simulink model "Brown_Control_Sim"  (R2025b)
settings: Solver=VariableStepAuto  StartTime=0.0  StopTime=10  RelTol=1e-3
undefined symbols (not defined in the file or in its folder): controller_airspeed_cmd_base, controller_airspeed_step, controller_bank_cmd_base, controller_bank_step, controller_enable, controller_front_motor_mask, controller_integrator_limit, controller_k_p_damp, controller_k_phi_i, controller_k_phi_p, controller_k_q_damp, controller_k_r_damp, controller_k_v_i, controller_k_v_p, controller_mode, controller_rpm_delta_limit, controller_sample_time, controller_step_time, controller_surface_limit_rad, controller_trim_delta_a, controller_trim_delta_e, controller_trim_delta_f, controller_trim_delta_r, controller_trim_motor_rpms, controller_trim_tilt_angles, estimator_enable, estimator_init_eul, estimator_k_acc, estimator_k_att, estimator_k_mag, estimator_sample_time, mag_ned, sensor_accel_bias, sensor_accel_sigma, sensor_airdata_bias, sensor_airdata_sigma, sensor_attitude_bias, sensor_attitude_sigma, sensor_enable_bias, sensor_enable_noise, sensor_gps_pos_bias, sensor_gps_pos_sigma, sensor_gps_vel_bias, sensor_gps_vel_sigma, sensor_gyro_bias, sensor_gyro_sigma, sensor_mag_bias, sensor_mag_sigma, sensor_sample_time, trim_front_collective_rpm, trim_rear_collective_rpm
settings Model: Creator=zbrown  LastModifiedBy=zbrown

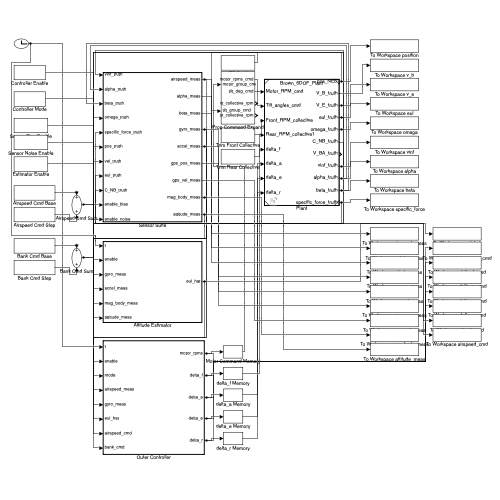
[thumbnail: Simulink's stored preview of the top-level diagram]
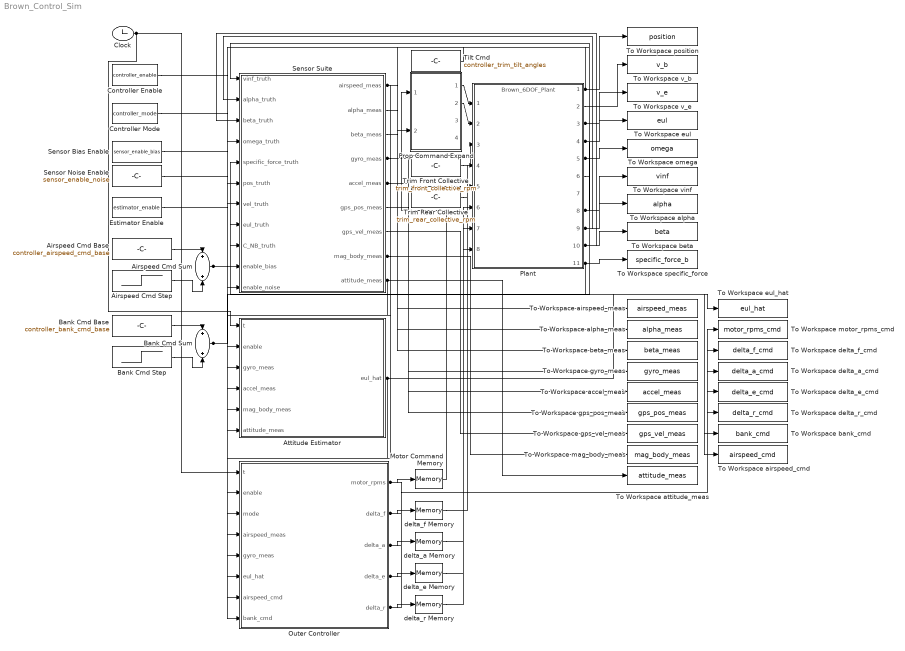
== system Brown_Control_Sim ==
  Airspeed Cmd Base : Constant  Value=controller_airspeed_cmd_base
  Airspeed Cmd Step : Step  Time=controller_step_time  After=controller_airspeed_step  SampleTime=0
  Airspeed Cmd Sum : Sum
  Attitude Estimator : Subsystem  TreatAsAtomicUnit=on  SystemSampleTime=estimator_sample_time
  Bank Cmd Base : Constant  Value=controller_bank_cmd_base
  Bank Cmd Step : Step  Time=controller_step_time  After=controller_bank_step  SampleTime=0
  Bank Cmd Sum : Sum
  Clock : Clock
  Controller Enable : Constant  Value=controller_enable
  Controller Mode : Constant  Value=controller_mode
  Estimator Enable : Constant  Value=estimator_enable
  Motor Command Memory : Memory
  Outer Controller : Subsystem  TreatAsAtomicUnit=on  SystemSampleTime=controller_sample_time
  Plant : ModelReference  ModelNameDialog=Brown_6DOF_Plant  SimulationMode=Normal  ModelReferenceVersion=1.27
  Prop Command Expand : Subsystem
  Sensor Bias Enable : Constant  Value=sensor_enable_bias
  Sensor Noise Enable : Constant  Value=sensor_enable_noise
  Sensor Suite : Subsystem  TreatAsAtomicUnit=on  SystemSampleTime=sensor_sample_time
  Tilt Cmd : Constant  Value=controller_trim_tilt_angles
  To Workspace accel_meas : ToWorkspace  VariableName=accel_meas  SampleTime=-1
  To Workspace airspeed_cmd : ToWorkspace  VariableName=airspeed_cmd  SampleTime=-1
  To Workspace airspeed_meas : ToWorkspace  VariableName=airspeed_meas  SampleTime=-1
  To Workspace alpha : ToWorkspace  VariableName=alpha  SampleTime=-1
  To Workspace alpha_meas : ToWorkspace  VariableName=alpha_meas  SampleTime=-1
  To Workspace attitude_meas : ToWorkspace  VariableName=attitude_meas  SampleTime=-1
  To Workspace bank_cmd : ToWorkspace  VariableName=bank_cmd  SampleTime=-1
  To Workspace beta : ToWorkspace  VariableName=beta  SampleTime=-1
  To Workspace beta_meas : ToWorkspace  VariableName=beta_meas  SampleTime=-1
  To Workspace delta_a_cmd : ToWorkspace  VariableName=delta_a_cmd  SampleTime=-1
  To Workspace delta_e_cmd : ToWorkspace  VariableName=delta_e_cmd  SampleTime=-1
  To Workspace delta_f_cmd : ToWorkspace  VariableName=delta_f_cmd  SampleTime=-1
  To Workspace delta_r_cmd : ToWorkspace  VariableName=delta_r_cmd  SampleTime=-1
  To Workspace eul : ToWorkspace  VariableName=eul  SampleTime=-1
  To Workspace eul_hat : ToWorkspace  VariableName=eul_hat  SampleTime=-1
  To Workspace gps_pos_meas : ToWorkspace  VariableName=gps_pos_meas  SampleTime=-1
  To Workspace gps_vel_meas : ToWorkspace  VariableName=gps_vel_meas  SampleTime=-1
  To Workspace gyro_meas : ToWorkspace  VariableName=gyro_meas  SampleTime=-1
  To Workspace mag_body_meas : ToWorkspace  VariableName=mag_body_meas  SampleTime=-1
  To Workspace motor_rpms_cmd : ToWorkspace  VariableName=motor_rpms_cmd  SampleTime=-1
  To Workspace omega : ToWorkspace  VariableName=omega  SampleTime=-1
  To Workspace position : ToWorkspace  VariableName=position  SampleTime=-1
  To Workspace specific_force : ToWorkspace  VariableName=specific_force_b  SampleTime=-1
  To Workspace v_b : ToWorkspace  VariableName=v_b  SampleTime=-1
  To Workspace v_e : ToWorkspace  VariableName=v_e  SampleTime=-1
  To Workspace vinf : ToWorkspace  VariableName=vinf  SampleTime=-1
  Trim Front Collective : Constant  Value=trim_front_collective_rpm
  Trim Rear Collective : Constant  Value=trim_rear_collective_rpm
  delta_a Memory : Memory
  delta_e Memory : Memory
  delta_f Memory : Memory
  delta_r Memory : Memory
  wires:
  Airspeed Cmd Base/1 -> Airspeed Cmd Sum/1
  Airspeed Cmd Step/1 -> Airspeed Cmd Sum/2
  Bank Cmd Base/1 -> Bank Cmd Sum/1
  Bank Cmd Step/1 -> Bank Cmd Sum/2
  Outer Controller/1(motor_rpms) -> Motor Command Memory/1, To Workspace motor_rpms_cmd/1
  Outer Controller/2(delta_f) -> delta_f Memory/1, To Workspace delta_f_cmd/1
  Outer Controller/3(delta_a) -> delta_a Memory/1, To Workspace delta_a_cmd/1
  Outer Controller/4(delta_e) -> delta_e Memory/1, To Workspace delta_e_cmd/1
  Outer Controller/5(delta_r) -> delta_r Memory/1, To Workspace delta_r_cmd/1
  Motor Command Memory/1 -> Prop Command Expand/1(motor_group_cmd)
  Tilt Cmd/1 -> Prop Command Expand/2(tilt_group_cmd)
  Prop Command Expand/1(motor_rpms_cmd) -> Plant/1
  Prop Command Expand/2(tilt_deg_cmd) -> Plant/2
  Trim Front Collective/1 -> Plant/3
  Trim Rear Collective/1 -> Plant/4
  delta_f Memory/1 -> Plant/5
  delta_a Memory/1 -> Plant/6
  delta_e Memory/1 -> Plant/7
  delta_r Memory/1 -> Plant/8
  Plant/8 -> Sensor Suite/1(vinf_truth), To Workspace vinf/1
  Plant/9 -> Sensor Suite/2(alpha_truth), To Workspace alpha/1
  Plant/10 -> Sensor Suite/3(beta_truth), To Workspace beta/1
  Plant/5 -> Sensor Suite/4(omega_truth), To Workspace omega/1
  Plant/11 -> Sensor Suite/5(specific_force_truth), To Workspace specific_force/1
  Plant/1 -> Sensor Suite/6(pos_truth), To Workspace position/1
  Plant/3 -> Sensor Suite/7(vel_truth), To Workspace v_e/1
  Plant/4 -> Sensor Suite/8(eul_truth), To Workspace eul/1
  Plant/6 -> Sensor Suite/9(C_NB_truth)
  Sensor Bias Enable/1 -> Sensor Suite/10(enable_bias)
  Sensor Noise Enable/1 -> Sensor Suite/11(enable_noise)
  Clock/1 -> Attitude Estimator/1(t), Outer Controller/1(t)
  Estimator Enable/1 -> Attitude Estimator/2(enable)
  Sensor Suite/4(gyro_meas) -> Attitude Estimator/3(gyro_meas), Outer Controller/5(gyro_meas), To Workspace gyro_meas/1
  Sensor Suite/5(accel_meas) -> Attitude Estimator/4(accel_meas), To Workspace accel_meas/1
  Sensor Suite/8(mag_body_meas) -> Attitude Estimator/5(mag_body_meas), To Workspace mag_body_meas/1
  Sensor Suite/9(attitude_meas) -> Attitude Estimator/6(attitude_meas), To Workspace attitude_meas/1
  Controller Enable/1 -> Outer Controller/2(enable)
  Controller Mode/1 -> Outer Controller/3(mode)
  Sensor Suite/1(airspeed_meas) -> Outer Controller/4(airspeed_meas), To Workspace airspeed_meas/1
  Attitude Estimator/1(eul_hat) -> Outer Controller/6(eul_hat), To Workspace eul_hat/1
  Airspeed Cmd Sum/1 -> Outer Controller/7(airspeed_cmd), To Workspace airspeed_cmd/1
  Bank Cmd Sum/1 -> Outer Controller/8(bank_cmd), To Workspace bank_cmd/1
  Plant/2 -> To Workspace v_b/1
  Sensor Suite/2(alpha_meas) -> To Workspace alpha_meas/1
  Sensor Suite/3(beta_meas) -> To Workspace beta_meas/1
  Sensor Suite/6(gps_pos_meas) -> To Workspace gps_pos_meas/1
  Sensor Suite/7(gps_vel_meas) -> To Workspace gps_vel_meas/1

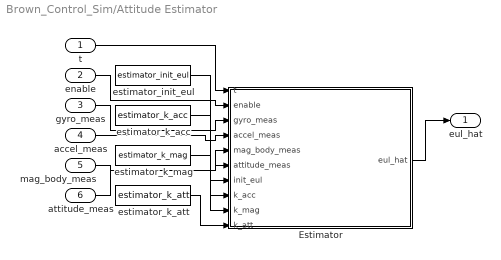
== system Brown_Control_Sim/Attitude Estimator ==
  t : Inport
  enable : Inport  Port=2
  gyro_meas : Inport  Port=3
  accel_meas : Inport  Port=4
  mag_body_meas : Inport  Port=5
  attitude_meas : Inport  Port=6
  Estimator : MATLAB Function  TreatAsAtomicUnit=on
  estimator_init_eul : Constant  Value=estimator_init_eul
  estimator_k_acc : Constant  Value=estimator_k_acc
  estimator_k_att : Constant  Value=estimator_k_att
  estimator_k_mag : Constant  Value=estimator_k_mag
  eul_hat : Outport
  wires:
  ? -> ?
  t/1 -> Estimator/1(t)
  enable/1 -> Estimator/2(enable)
  gyro_meas/1 -> Estimator/3(gyro_meas)
  accel_meas/1 -> Estimator/4(accel_meas)
  mag_body_meas/1 -> Estimator/5(mag_body_meas)
  attitude_meas/1 -> Estimator/6(attitude_meas)
  estimator_init_eul/1 -> Estimator/7(init_eul)
  estimator_k_acc/1 -> Estimator/8(k_acc)
  estimator_k_mag/1 -> Estimator/9(k_mag)
  estimator_k_att/1 -> Estimator/10(k_att)
  Estimator/1(eul_hat) -> eul_hat/1

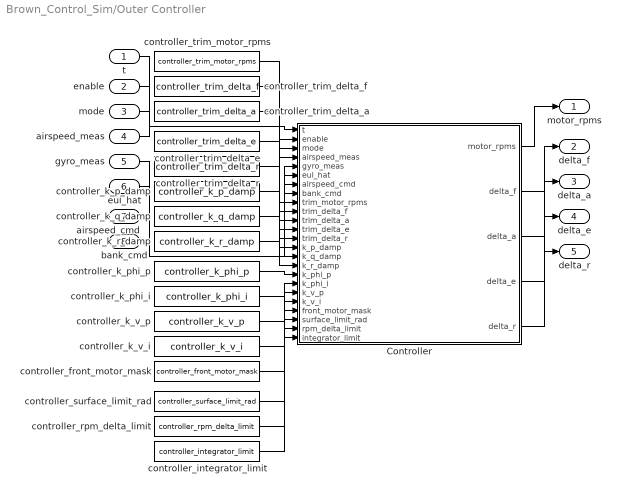
== system Brown_Control_Sim/Outer Controller ==
  t : Inport
  enable : Inport  Port=2
  mode : Inport  Port=3
  airspeed_meas : Inport  Port=4
  gyro_meas : Inport  Port=5
  eul_hat : Inport  Port=6
  airspeed_cmd : Inport  Port=7
  bank_cmd : Inport  Port=8
  Controller : MATLAB Function  TreatAsAtomicUnit=on
  controller_front_motor_mask : Constant  Value=controller_front_motor_mask
  controller_integrator_limit : Constant  Value=controller_integrator_limit
  controller_k_p_damp : Constant  Value=controller_k_p_damp
  controller_k_phi_i : Constant  Value=controller_k_phi_i
  controller_k_phi_p : Constant  Value=controller_k_phi_p
  controller_k_q_damp : Constant  Value=controller_k_q_damp
  controller_k_r_damp : Constant  Value=controller_k_r_damp
  controller_k_v_i : Constant  Value=controller_k_v_i
  controller_k_v_p : Constant  Value=controller_k_v_p
  controller_rpm_delta_limit : Constant  Value=controller_rpm_delta_limit
  controller_surface_limit_rad : Constant  Value=controller_surface_limit_rad
  controller_trim_delta_a : Constant  Value=controller_trim_delta_a
  controller_trim_delta_e : Constant  Value=controller_trim_delta_e
  controller_trim_delta_f : Constant  Value=controller_trim_delta_f
  controller_trim_delta_r : Constant  Value=controller_trim_delta_r
  controller_trim_motor_rpms : Constant  Value=controller_trim_motor_rpms
  motor_rpms : Outport
  delta_f : Outport  Port=2
  delta_a : Outport  Port=3
  delta_e : Outport  Port=4
  delta_r : Outport  Port=5
  wires:
  ? -> ?
  t/1 -> Controller/1(t)
  enable/1 -> Controller/2(enable)
  mode/1 -> Controller/3(mode)
  airspeed_meas/1 -> Controller/4(airspeed_meas)
  gyro_meas/1 -> Controller/5(gyro_meas)
  eul_hat/1 -> Controller/6(eul_hat)
  airspeed_cmd/1 -> Controller/7(airspeed_cmd)
  bank_cmd/1 -> Controller/8(bank_cmd)
  controller_trim_motor_rpms/1 -> Controller/9(trim_motor_rpms)
  controller_trim_delta_f/1 -> Controller/10(trim_delta_f)
  controller_trim_delta_a/1 -> Controller/11(trim_delta_a)
  controller_trim_delta_e/1 -> Controller/12(trim_delta_e)
  controller_trim_delta_r/1 -> Controller/13(trim_delta_r)
  controller_k_p_damp/1 -> Controller/14(k_p_damp)
  controller_k_q_damp/1 -> Controller/15(k_q_damp)
  controller_k_r_damp/1 -> Controller/16(k_r_damp)
  controller_k_phi_p/1 -> Controller/17(k_phi_p)
  controller_k_phi_i/1 -> Controller/18(k_phi_i)
  controller_k_v_p/1 -> Controller/19(k_v_p)
  controller_k_v_i/1 -> Controller/20(k_v_i)
  controller_front_motor_mask/1 -> Controller/21(front_motor_mask)
  controller_surface_limit_rad/1 -> Controller/22(surface_limit_rad)
  controller_rpm_delta_limit/1 -> Controller/23(rpm_delta_limit)
  controller_integrator_limit/1 -> Controller/24(integrator_limit)
  Controller/1(motor_rpms) -> motor_rpms/1
  Controller/2(delta_f) -> delta_f/1
  Controller/3(delta_a) -> delta_a/1
  Controller/4(delta_e) -> delta_e/1
  Controller/5(delta_r) -> delta_r/1

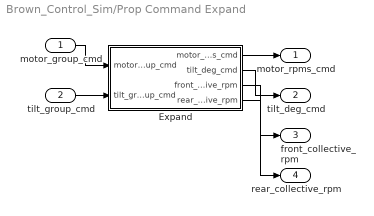
== system Brown_Control_Sim/Prop Command Expand ==
  motor_group_cmd : Inport
  tilt_group_cmd : Inport  Port=2
  Expand : MATLAB Function  TreatAsAtomicUnit=on
  motor_rpms_cmd : Outport
  tilt_deg_cmd : Outport  Port=2
  front_collective_rpm : Outport  Port=3
  rear_collective_rpm : Outport  Port=4
  wires:
  ? -> ?
  motor_group_cmd/1 -> Expand/1(motor_group_cmd)
  tilt_group_cmd/1 -> Expand/2(tilt_group_cmd)
  Expand/1(motor_rpms_cmd) -> motor_rpms_cmd/1
  Expand/2(tilt_deg_cmd) -> tilt_deg_cmd/1
  Expand/3(front_collective_rpm) -> front_collective_rpm/1
  Expand/4(rear_collective_rpm) -> rear_collective_rpm/1

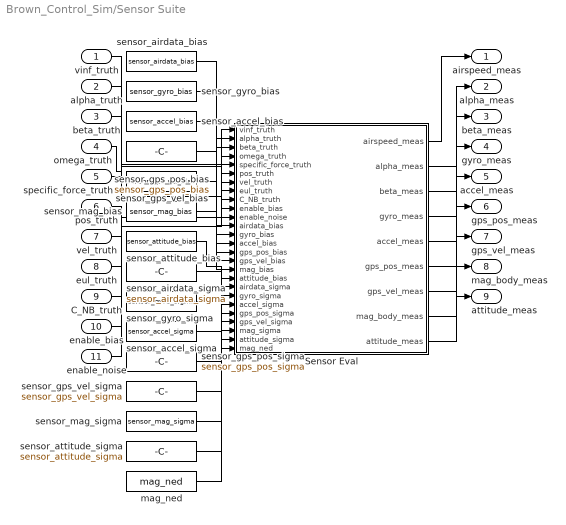
== system Brown_Control_Sim/Sensor Suite ==
  vinf_truth : Inport
  alpha_truth : Inport  Port=2
  beta_truth : Inport  Port=3
  omega_truth : Inport  Port=4
  specific_force_truth : Inport  Port=5
  pos_truth : Inport  Port=6
  vel_truth : Inport  Port=7
  eul_truth : Inport  Port=8
  C_NB_truth : Inport  Port=9
  enable_bias : Inport  Port=10
  enable_noise : Inport  Port=11
  Sensor Eval : MATLAB Function  TreatAsAtomicUnit=on
  mag_ned : Constant  Value=mag_ned
  sensor_accel_bias : Constant  Value=sensor_accel_bias
  sensor_accel_sigma : Constant  Value=sensor_accel_sigma
  sensor_airdata_bias : Constant  Value=sensor_airdata_bias
  sensor_airdata_sigma : Constant  Value=sensor_airdata_sigma
  sensor_attitude_bias : Constant  Value=sensor_attitude_bias
  sensor_attitude_sigma : Constant  Value=sensor_attitude_sigma
  sensor_gps_pos_bias : Constant  Value=sensor_gps_pos_bias
  sensor_gps_pos_sigma : Constant  Value=sensor_gps_pos_sigma
  sensor_gps_vel_bias : Constant  Value=sensor_gps_vel_bias
  sensor_gps_vel_sigma : Constant  Value=sensor_gps_vel_sigma
  sensor_gyro_bias : Constant  Value=sensor_gyro_bias
  sensor_gyro_sigma : Constant  Value=sensor_gyro_sigma
  sensor_mag_bias : Constant  Value=sensor_mag_bias
  sensor_mag_sigma : Constant  Value=sensor_mag_sigma
  airspeed_meas : Outport
  alpha_meas : Outport  Port=2
  beta_meas : Outport  Port=3
  gyro_meas : Outport  Port=4
  accel_meas : Outport  Port=5
  gps_pos_meas : Outport  Port=6
  gps_vel_meas : Outport  Port=7
  mag_body_meas : Outport  Port=8
  attitude_meas : Outport  Port=9
  wires:
  ? -> ?
  vinf_truth/1 -> Sensor Eval/1(vinf_truth)
  alpha_truth/1 -> Sensor Eval/2(alpha_truth)
  beta_truth/1 -> Sensor Eval/3(beta_truth)
  omega_truth/1 -> Sensor Eval/4(omega_truth)
  specific_force_truth/1 -> Sensor Eval/5(specific_force_truth)
  pos_truth/1 -> Sensor Eval/6(pos_truth)
  vel_truth/1 -> Sensor Eval/7(vel_truth)
  eul_truth/1 -> Sensor Eval/8(eul_truth)
  C_NB_truth/1 -> Sensor Eval/9(C_NB_truth)
  enable_bias/1 -> Sensor Eval/10(enable_bias)
  enable_noise/1 -> Sensor Eval/11(enable_noise)
  sensor_airdata_bias/1 -> Sensor Eval/12(airdata_bias)
  sensor_gyro_bias/1 -> Sensor Eval/13(gyro_bias)
  sensor_accel_bias/1 -> Sensor Eval/14(accel_bias)
  sensor_gps_pos_bias/1 -> Sensor Eval/15(gps_pos_bias)
  sensor_gps_vel_bias/1 -> Sensor Eval/16(gps_vel_bias)
  sensor_mag_bias/1 -> Sensor Eval/17(mag_bias)
  sensor_attitude_bias/1 -> Sensor Eval/18(attitude_bias)
  sensor_airdata_sigma/1 -> Sensor Eval/19(airdata_sigma)
  sensor_gyro_sigma/1 -> Sensor Eval/20(gyro_sigma)
  sensor_accel_sigma/1 -> Sensor Eval/21(accel_sigma)
  sensor_gps_pos_sigma/1 -> Sensor Eval/22(gps_pos_sigma)
  sensor_gps_vel_sigma/1 -> Sensor Eval/23(gps_vel_sigma)
  sensor_mag_sigma/1 -> Sensor Eval/24(mag_sigma)
  sensor_attitude_sigma/1 -> Sensor Eval/25(attitude_sigma)
  mag_ned/1 -> Sensor Eval/26(mag_ned)
  Sensor Eval/1(airspeed_meas) -> airspeed_meas/1
  Sensor Eval/2(alpha_meas) -> alpha_meas/1
  Sensor Eval/3(beta_meas) -> beta_meas/1
  Sensor Eval/4(gyro_meas) -> gyro_meas/1
  Sensor Eval/5(accel_meas) -> accel_meas/1
  Sensor Eval/6(gps_pos_meas) -> gps_pos_meas/1
  Sensor Eval/7(gps_vel_meas) -> gps_vel_meas/1
  Sensor Eval/8(mag_body_meas) -> mag_body_meas/1
  Sensor Eval/9(attitude_meas) -> attitude_meas/1

== matlab function Brown_Control_Sim/Prop Command Expand/Expand ==
  data: motor_group_cmd input; motor_rpms_cmd output; tilt_group_cmd input; tilt_deg_cmd output; front_collective_rpm output; rear_collective_rpm output
function [motor_rpms_cmd, tilt_deg_cmd, front_collective_rpm, rear_collective_rpm] = fcn(motor_group_cmd, tilt_group_cmd)
%#codegen
fr = motor_group_cmd(1);
fl = motor_group_cmd(2);
rr = motor_group_cmd(3);
rl = motor_group_cmd(4);
motor_rpms_cmd = [fr; fr; fr; fl; fl; fl; rr; rr; rr; rl; rl; rl];
tilt_fr = tilt_group_cmd(1);
tilt_fl = tilt_group_cmd(2);
tilt_deg_cmd = [tilt_fr; tilt_fr; tilt_fr; tilt_fl; tilt_fl; tilt_fl];
front_collective_rpm = 0.5 * (fr + fl);
rear_collective_rpm = 0.5 * (rr + rl);
end

== matlab function Brown_Control_Sim/Attitude Estimator/Estimator ==
  data: t input; eul_hat output; enable input; gyro_meas input; accel_meas input; mag_body_meas input; attitude_meas input; init_eul input; k_acc input; k_mag input; k_att input
function eul_hat = fcn(t, enable, gyro_meas, accel_meas, mag_body_meas, attitude_meas, init_eul, k_acc, k_mag, k_att)
%#codegen
eul_hat = attitude_complementary_step(t, enable, gyro_meas, accel_meas, mag_body_meas, attitude_meas, init_eul, k_acc, k_mag, k_att);
end

== matlab function Brown_Control_Sim/Sensor Suite/Sensor Eval ==
  data: vinf_truth input; airspeed_meas output; alpha_truth input; beta_truth input; omega_truth input; specific_force_truth input; pos_truth input; vel_truth input; eul_truth input; C_NB_truth input; enable_bias input; enable_noise input; airdata_bias input; gyro_bias input; accel_bias input; gps_pos_bias input; gps_vel_bias input; mag_bias input; attitude_bias input; airdata_sigma input; gyro_sigma input; accel_sigma input; gps_pos_sigma input; gps_vel_sigma input; mag_sigma input; attitude_sigma input; mag_ned input; alpha_meas output; beta_meas output; gyro_meas output; accel_meas output; gps_pos_meas output; gps_vel_meas output; mag_body_meas output; attitude_meas output
function [airspeed_meas, alpha_meas, beta_meas, gyro_meas, accel_meas, gps_pos_meas, gps_vel_meas, mag_body_meas, attitude_meas] = fcn(vinf_truth, alpha_truth, beta_truth, omega_truth, specific_force_truth, pos_truth, vel_truth, eul_truth, C_NB_truth, enable_bias, enable_noise, airdata_bias, gyro_bias, accel_bias, gps_pos_bias, gps_vel_bias, mag_bias, attitude_bias, airdata_sigma, gyro_sigma, accel_sigma, gps_pos_sigma, gps_vel_sigma, mag_sigma, attitude_sigma, mag_ned)
%#codegen
[airspeed_meas, alpha_meas, beta_meas, gyro_meas, accel_meas, gps_pos_meas, gps_vel_meas, mag_body_meas, attitude_meas] = sensor_suite_eval(vinf_truth, alpha_truth, beta_truth, omega_truth, specific_force_truth, pos_truth, vel_truth, eul_truth, C_NB_truth, enable_bias, enable_noise, airdata_bias, gyro_bias, accel_bias, gps_pos_bias, gps_vel_bias, mag_bias, attitude_bias, airdata_sigma, gyro_sigma, accel_sigma, gps_pos_sigma, gps_vel_sigma, mag_sigma, attitude_sigma, mag_ned);
end

== matlab function Brown_Control_Sim/Outer Controller/Controller ==
  data: t input; motor_rpms output; enable input; mode input; airspeed_meas input; gyro_meas input; eul_hat input; airspeed_cmd input; bank_cmd input; trim_motor_rpms input; trim_delta_f input; trim_delta_a input; trim_delta_e input; trim_delta_r input; k_p_damp input; k_q_damp input; k_r_damp input; k_phi_p input; k_phi_i input; k_v_p input; k_v_i input; front_motor_mask input; surface_limit_rad input; rpm_delta_limit input; integrator_limit input; delta_f output; delta_a output; delta_e output; delta_r output
function [motor_rpms, delta_f, delta_a, delta_e, delta_r] = fcn(t, enable, mode, airspeed_meas, gyro_meas, eul_hat, airspeed_cmd, bank_cmd, trim_motor_rpms, trim_delta_f, trim_delta_a, trim_delta_e, trim_delta_r, k_p_damp, k_q_damp, k_r_damp, k_phi_p, k_phi_i, k_v_p, k_v_i, front_motor_mask, surface_limit_rad, rpm_delta_limit, integrator_limit)
%#codegen
[motor_rpms, delta_f, delta_a, delta_e, delta_r] = outer_controller_step(t, enable, mode, airspeed_meas, gyro_meas, eul_hat, airspeed_cmd, bank_cmd, trim_motor_rpms, trim_delta_f, trim_delta_a, trim_delta_e, trim_delta_r, k_p_damp, k_q_damp, k_r_damp, k_phi_p, k_phi_i, k_v_p, k_v_i, front_motor_mask, surface_limit_rad, rpm_delta_limit, integrator_limit);
end
